simulink model "LAB06"  (R2023b)
settings: Solver=VariableStepAuto  StartTime=0.0  StopTime=15  RelTol=1e-3
libraries: spsDCVoltageSourceLib x2, spsDCMachineLib x1, sps_lib x1
settings Model: Creator=sanju  LastModifiedBy=sagar

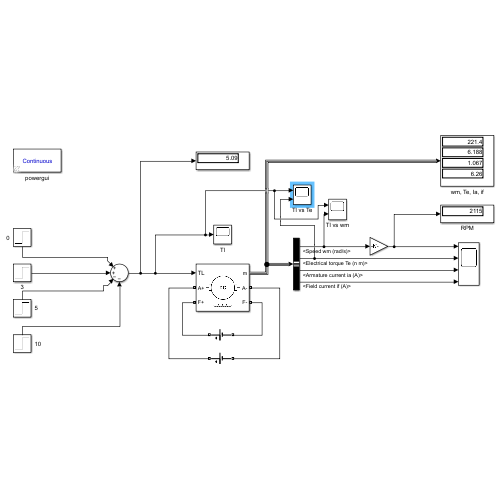
[thumbnail: Simulink's stored preview of the top-level diagram]
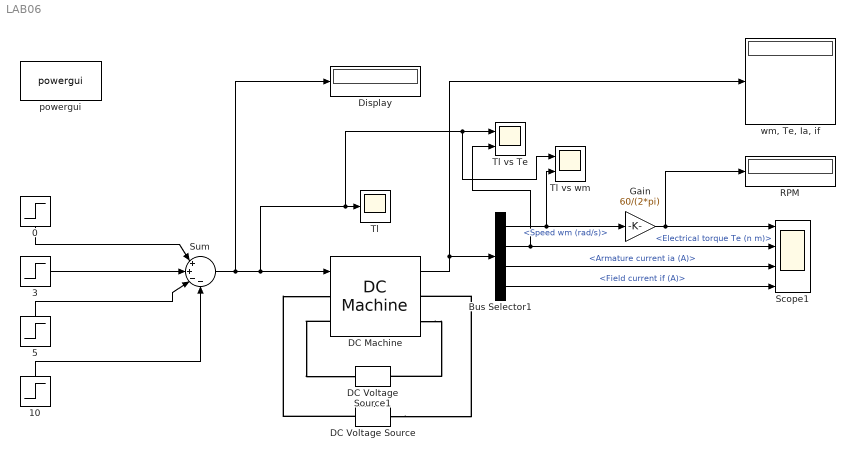
== system LAB06 ==
  0 : Step  Time=0  After=0  SampleTime=0
  10 : Step  Time=10  After=5.09  SampleTime=0
  3 : Step  Time=3  After=20.36  SampleTime=0
  5 : Step  Time=5  After=10.18  SampleTime=0
  Bus Selector1 : BusSelector  OutputSignals=Speed wm (rad/s),Electrical torque Te (n m),Armature current ia (A),Field current if (A)
  DC Machine : spsDCMachineLib/DC Machine  PresetModel=01: 5HP 240V 1750RPM Field:300V  MechanicalLoad=Torque TL  FieldType=Wound  ShowDetailedParameters=on  MeasurementBus=off  RLa=[2.581 0.028]  RLf=[281.2 156]  Laf=0.9483  MachineConstant=Torque constant (N.m/A)  Ke=1.8  Kt=1.8  J=0.02215  Bm=0.002953  Tf=0.5161  w0=1  Ifinit=1.06685633001422  TsPowergui=0  TsBlock=-1
  DC Voltage Source : spsDCVoltageSourceLib/DC Voltage Source  Amplitude=240  Measurements=None
  DC Voltage Source1 : spsDCVoltageSourceLib/DC Voltage Source  Amplitude=300  Measurements=None
  Display : Display
  Gain : Gain  Gain=60/(2*pi)
  RPM : Display
  Scope1 : Scope  NumInputPorts=4
  Sum : Sum  Inputs=|++--
  Tl : Scope
  Tl vs Te : Scope  NumInputPorts=2
  Tl vs wm : Scope  NumInputPorts=2
  powergui : sps_lib/powergui  Priority=1  SimulationMode=Continuous  SampleTime=50e-6  frequency=60  Iterations=50  frequencyindice=0  Pbase=100e6  ErrMax=1e-4  UnitsV=kV  UnitsW=MW  buscounter=0  FunctionMessages=off  echomessages=off  EnableUseOfTLC=off  CurrentSourceSwitches=off  DisableSnubberDevices=off  DisableRonSwitches=off  DisableVfSwitches=off  DisplayEquations=off  AutomaticDiscreteSolvers=off  SolverType=Tustin/Backward Euler (TBE)  Interpol=off  ExternalGateDelay=off  methode=off  Ts=100  x0status=blocks  SPID=on  SwTol=0  HookPort=off  NonlinearTolerance=1e-4  nMaxIteration=100  ContinueOnMaxIteration=off  RestoreLinks=warning  ResistiveCurrentMeasurement=off  Frange=[0:2:500]  Ylog=off  Xlog=on  ShowGrid=off  save=off  variable=ZData  structure=0  ZoomFFT=off  StartTime=0.0  cycles=1  DisplayStyle=1  fundamental=60  FreqAxis=off  MaxFrequency=1000  frequencyindicesteady=1  RmsSteady=1  display=off
  "wm, Te, Ia, if" : Display
  wires:
  Sum/1 -> Tl vs wm/1, Tl vs Te/1, Tl/1, DC Machine/1, Display/1
  DC Machine/1 -> "wm, Te, Ia, if"/1, Bus Selector1/1
  3/1 -> Sum/2
  5/1 -> Sum/3
  0/1 -> Sum/1
  Bus Selector1/1 -> Gain/1, Tl vs wm/2  "<Speed wm (rad/s)>"
  Bus Selector1/4 -> Scope1/4  "<Field current if (A)>"
  Bus Selector1/3 -> Scope1/3  "<Armature current ia (A)>"
  Bus Selector1/2 -> Tl vs Te/2, Scope1/2  "<Electrical torque Te (n m)>"
  10/1 -> Sum/4
  Gain/1 -> RPM/1, Scope1/1
  connections:
  DC Machine/LConn2 -- DC Voltage Source1/RConn1
  DC Machine/RConn2 -- DC Voltage Source1/LConn1
  DC Voltage Source/RConn1 -- DC Machine/LConn1
  DC Voltage Source/LConn1 -- DC Machine/RConn1
